simulink model "HW6prob2a"  (Simulink 7.8)
settings: Solver=ode45  StartTime=0.0  StopTime=6  RelTol=1e-3
values from neighbouring files (symbols this model uses):
  A = [0, 1; -2, -3]    [16-31-hw-6.m]
  B = [0; 1]    [16-31-hw-6.m]
  K = Kb    [16-31-hw-6.m]
  uncert = 0.1    [16-31-hw-6.m]
settings Model: Creator=Dan  LastModifiedBy=Dan

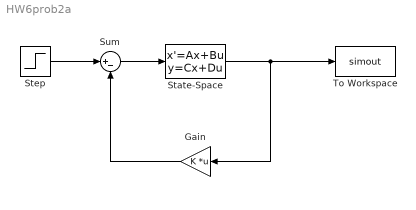
== system HW6prob2a ==
  Gain : Gain  Gain=K  Multiplication=Matrix(K*u)
  State-Space : StateSpace  A=A+eye(2,2)*uncert  B=B  C=eye(2,2)  D=[0;0]
  Step : Step  SampleTime=0
  Sum : Sum  Inputs=|+-
  To Workspace : ToWorkspace  VariableName=simout  SampleTime=-1  SaveFormat=Structure
  wires:
  Gain/1 -> Sum/2
  Step/1 -> Sum/1
  Sum/1 -> State-Space/1
  State-Space/1 -> Gain/1, To Workspace/1
